simulink model "Kronecker_Ex2"  (R2025a)
settings: Solver=VariableStepAuto  StartTime=0.0  StopTime=100  RelTol=1e-3
undefined symbols (not defined in the file): Correlation_ValidMode, DUT, L, vsva1596, xcvc1702
libraries: aieUtilities x2, aieDSP x1, vmcUtilities x1
settings Model: Creator=sdegala  LastModifiedBy=sdegala
settings ModelReferenceCC: EnableRefExpFcnMdlSchedulingChecks=on
settings RTWCC: GPUComputeCapability=3.5

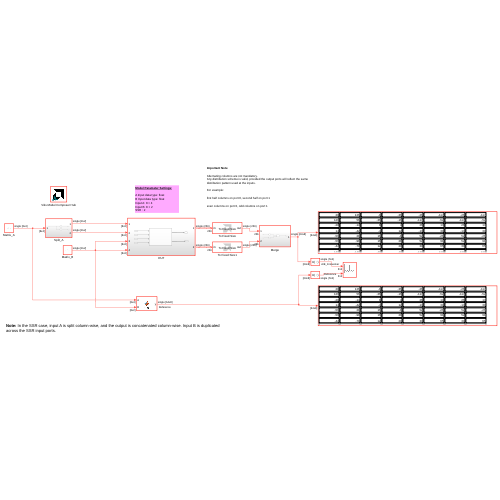
[thumbnail: Simulink's stored preview of the top-level diagram]
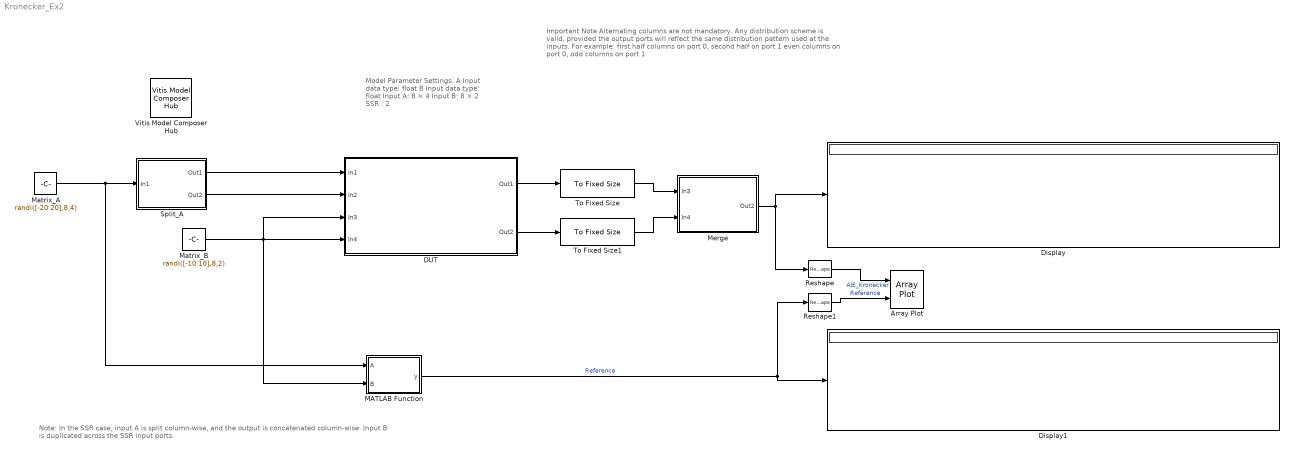
== system Kronecker_Ex2 ==
  note: Important Note
      |
      | Alternating columns are not mandatory.
      | Any distribution scheme is valid, provided the output ports will reflect the same distribution pattern used at the inputs.
      |
      | For example:
      |
      | first half columns on port 0, second half on port 1
      |
      | even columns on port 0, odd columns on port 1
  note: Note: In the SSR case, input A is split column-wise, and the output is concatenated column-wise. Input B is duplicated across the SSR input ports.
  note: Model Parameter Settings:
      |
      | A Input data type: float
      | B Input data type: float
      | Input A: 8 × 4
      | Input B: 8 × 2
      | SSR : 2
  Array Plot : ArrayPlot  NumInputPorts=2  WindowPosition=[560.000000,350.000000,800.000000,500.000000,]  Visible=on  ScopeFrameLocation=window  YLimits=[-250 250]  ShowLegend=on
  DUT : Subsystem
  Display : Display
  Display1 : Display
  MATLAB Function : MATLAB Function  TreatAsAtomicUnit=on
  Matrix_A : Constant  Value=randi([-20 20],8,4)  OutDataTypeStr=single  SampleTime=1
  Matrix_B : Constant  Value=randi([-10 10],8,2)  OutDataTypeStr=single  SampleTime=1
  Merge : Subsystem
  Reshape : Reshape
  Reshape1 : Reshape
  Split_A : Subsystem
  To Fixed Size : aieUtilities/To Fixed Size  Mode=Stop simulation when input variable-size signal is not full  OutputSize=Inherit: Same as input  CopyMethod=Buffer samples to form output  HasStatusOutput=on
  To Fixed Size1 : aieUtilities/To Fixed Size  Mode=Stop simulation when input variable-size signal is not full  OutputSize=Inherit: Same as input  CopyMethod=Buffer samples to form output  HasStatusOutput=on
  Vitis Model Composer Hub : vmcUtilities/Vitis Model Composer Hub  Tag=genX  CodeGeneration=off  SubsystemName=DUT  BlockHierPath=Correlation_ValidMode/DUT  SubsystemType=AIENode  StartColumn=1  NumberOfColumns=1  TargetDirectory=./code  exportDesign=off  analyzeDesign=on  validateDesignOnHw=off  ExportType=AI Engines  IpVendor=xilinx.com  IpLibrary=hls  IpVersion=1.0  IpHWLanguage=Verilog  AieCompilerOptions={}  AieSimulatorOptions={}  AieGraphIterations=-1  CreateTestbench=on  TestbenchStackSize=10  RunRtlSim=off  RunCSim=off  RunAieSim=off  AieSimTimeout=50000  RunAieSimProfiling=off  LaunchVitisAnalyzer=off  PlotOutput=off  RunX86Sim=off  X86SimTimeout=10  GenHwImage=off  GenLibadfXo=off  GenHwValidationCode=off  PlatformType=Not Specified  HwSystemType=Baremetal  HwValidationTarget=hw  ProjDevice=xcvc1702-vsva1596-2LP-e-L  ProjDevicePart=xcvc1702-vsva1596-2LP-e-L  AIEType=AIE  SamplePeriod=-1  ClockFrequency=200  DataPathParallelism=1  xilinxfamily=versalaicore  part=xcvc1702  speed=-2LP-e-L  package=vsva1596  directory=./netlist  testbench=off  incr_netlist=off  synthesis_tool=Vivado  clock_wrapper=Clock Enables  dbl_ovrd=According to Block Masks  dcm_input_clock_period=10  sysclk_period=10  simulink_period=1  eval_field=0  IPInfoJsonString="{\"DUTSubsystemName\":\"DUT\",\"AIESubsystem\":{\"SubsystemName\":\"DUT\",\"TargetDirectory\":\"./code\",\"AIEArrayConfig\":\"Use entire AIE array\",\"StartColumn\":\"0\",\"NumberOfColumns\":\"1\"},\"SubsystemTag\":\"AIENode\"}"  LogFileName=/proj/xhdhdstaff5/sdegala/Head1/HEAD/2025_2_work/AIE_BLOCKS_2025_2/code/model_composer.log  NThreads=4  IPConfigFile=/tmp/vmctmp-11198269997411262707/Correlation_ValidMode_ipconfig.json
  wires:
  Matrix_A/1 -> MATLAB Function/1(A), Split_A/1(In1)
  Split_A/1(Out1) -> DUT/1(In1)
  Split_A/2(Out2) -> DUT/2(In2)
  Matrix_B/1 -> MATLAB Function/2(B), DUT/4(In4), DUT/3(In3)
  MATLAB Function/1(y) -> Reshape1/1, Display1/1  "Reference"
  DUT/1(Out1) -> To Fixed Size/1
  To Fixed Size/1 -> Merge/1(In3)
  DUT/2(Out2) -> To Fixed Size1/1
  To Fixed Size1/1 -> Merge/2(In4)
  Merge/1(Out2) -> Display/1, Reshape/1
  Reshape/1 -> Array Plot/1  "AIE_Kronecker"
  Reshape1/1 -> Array Plot/2  "Reference"

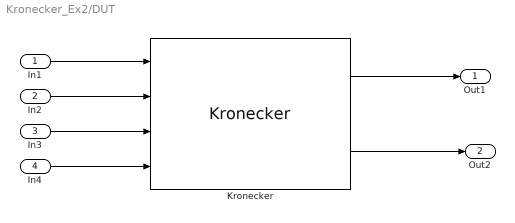
== system Kronecker_Ex2/DUT ==
  In1 : Inport
  In2 : Inport  Port=2
  In3 : Inport  Port=3
  In4 : Inport  Port=4
  Kronecker : aieDSP/Kronecker  AIE_VARIANT=1  TP_API=0  data_type_A=float  data_type_B=float  dim_a_rows=8  dim_a_cols=4  dim_b_rows=8  dim_b_cols=2  num_frames=1  shift_output=0  ssr=2  rnd_mode=Floor  sat_mode=None  blockJsonConstraints=[]  blockJsonConstraintsInternal=[]  spec=vmc_kronecker.json  SerializedMaskParamNames=[]  SerializedMaskParamValues=[]  SerializedMaskParamVisibilities=[]  block_type=Kronecker  SerializedMaskParamDataypes=uint|uint|typename|typename|uint|uint|uint|uint|uint|uint|uint|uint|uint  SerializedMaskParamEnumStrArr=0|0|0|0|0|0|0|0|0|0|0|Floor,Ceiling,Round to positive infinity,Round to negative infinity,Round symmetrical to infinity,Round symmetrical to zero,Round convergent to even,Round convergent to odd|None,Saturate,Symmetric  SerializedMaskParamEnumValArr=0|0|0|0|0|0|0|0|0|0|0|0,1,2,3,4,5,6,7|0,1,3  SerializedMaskParamVectorArr=0|0|0|0|0|0|0|0|0|0|0|0|0  SerializedMaskParamKeys=AIE_VARIANT|TP_API|TT_DATA_A|TT_DATA_B|TP_DIM_A_ROWS|TP_DIM_A_COLS|TP_DIM_B_ROWS|TP_DIM_B_COLS|TP_NUM_FRAMES|TP_SHIFT|TP_SSR|TP_RND|TP_SAT
  Out1 : Outport
  Out2 : Outport  Port=2
  wires:
  In1/1 -> Kronecker/1
  In2/1 -> Kronecker/2
  Kronecker/2 -> Out2/1
  In4/1 -> Kronecker/4
  Kronecker/1 -> Out1/1
  In3/1 -> Kronecker/3

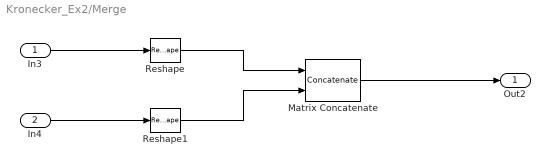
== system Kronecker_Ex2/Merge ==
  In3 : Inport
  In4 : Inport  Port=2
  Matrix Concatenate : Concatenate  Mode=Multidimensional array  ConcatenateDimension=2
  Reshape : Reshape  OutputDimensionality=Customize  OutputDimensions=[64,4]
  Reshape1 : Reshape  OutputDimensionality=Customize  OutputDimensions=[64,4]
  Out2 : Outport
  wires:
  In3/1 -> Reshape/1
  In4/1 -> Reshape1/1
  Reshape/1 -> Matrix Concatenate/1
  Reshape1/1 -> Matrix Concatenate/2
  Matrix Concatenate/1 -> Out2/1

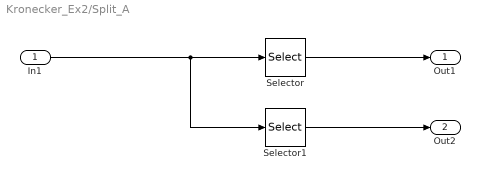
== system Kronecker_Ex2/Split_A ==
  In1 : Inport
  Selector : Selector  NumberOfDimensions=2  InputPortWidth=64  IndexOptions=Index vector (dialog),Index vector (dialog)  Indices=1:1:8,1:1:2  OutputSizes=1,1
  Selector1 : Selector  NumberOfDimensions=2  InputPortWidth=64  IndexOptions=Index vector (dialog),Index vector (dialog)  Indices=1:1:8,3:1:4  OutputSizes=1,1
  Out1 : Outport
  Out2 : Outport  Port=2
  wires:
  In1/1 -> Selector/1, Selector1/1
  Selector1/1 -> Out2/1
  Selector/1 -> Out1/1

== matlab function Kronecker_Ex2/MATLAB Function ==
  data: A input; y output; B input
 function y = fcn(A,B)
  y = kron(A,B);
